simulink model "GNSS_INS"  (R2019b)
settings: Solver=ode3  StartTime=0.0  StopTime=60.0  FixedStep=0.01  RelTol=1e-3
PreLoadFcn:
  | %% SETUP
  | % Start or connect to ROS master
  | rosshutdown;
  | rosinit()
undefined symbols (not defined in the file): Pose, Twist
libraries: robotlib x5
settings Model: Creator=adity  LastModifiedBy=adity
settings OptimizationCC: EnhancedBackFolding=on  PassReuseOutputArgsAs=Individual arguments  ZeroExternalMemoryAtStartup=off  ZeroInternalMemoryAtStartup=off  MaxStackSize=64  OptimizeBlockOrder=speed  DifferentSizesBufferReuse=on  OptimizationCustomize=off  EfficientTunableParamExpr=on
settings DebuggingCC: ParameterTunabilityLossMsg=error
settings HardwareCC: ProdBitPerPointer=32  ProdBitPerSizeT=32  ProdBitPerPtrDiffT=32  ProdLargestAtomicFloat=None  ProdIntDivRoundTo=Undefined  ProdEndianess=Unspecified  ProdWordSize=32  ProdHWDeviceType=Generic->Unspecified (assume 32-bit Generic)  UseEmbeddedCoderFeatures=off
settings SFSimCC: MATLABDynamicMemAlloc=off
settings RTWCC: SystemTargetFile=ert.tlc  HardwareBoard=Robot Operating System (ROS)  TLCOptions="-aInlineSetEventsForThisBaseRateFcn=TLC_FALSE -aSuppressMultiTaskScheduler=TLC_FALSE  -aRateBasedStepFcn=0"  TemplateMakefile=ert_default_tmf  GenerateReport=on  Toolchain=Catkin  IncludeHyperlinkInReport=on  LaunchReport=on  TargetLang=C++  GenerateTraceInfo=on  GenerateTraceReport=on  GenerateTraceReportSl=on  GenerateTraceReportSf=on  GenerateTraceReportEml=on
settings CodeAppCC: ForceParamTrailComments=on  IgnoreCustomStorageClasses=off  OperatorAnnotations=on  SimulinkDataObjDesc=on  SFDataObjDesc=on  InsertBlockDesc=on
settings ERTTargetCC: SupportNonInlinedSFcns=on

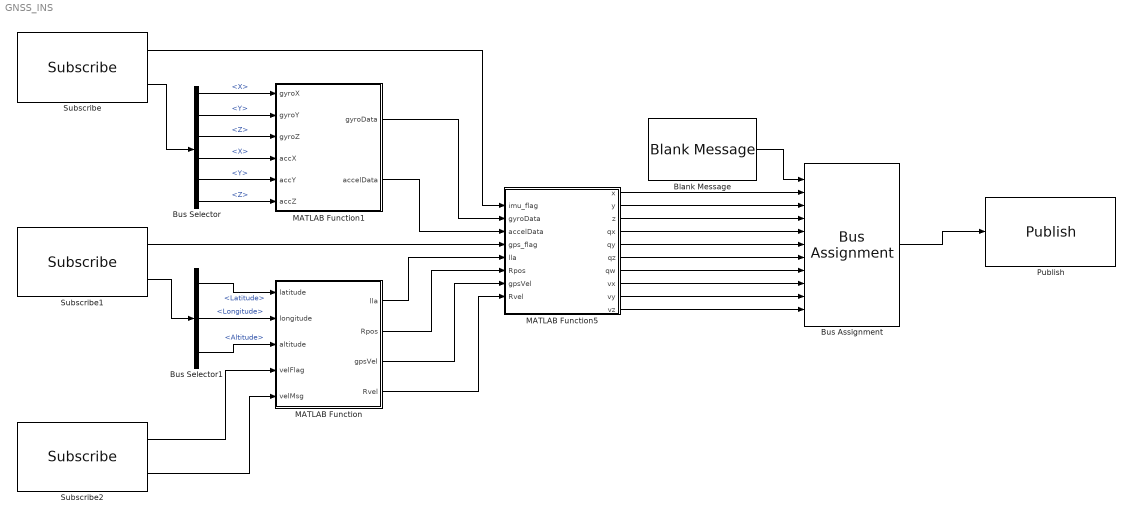
== system GNSS_INS ==
  Blank Message : robotlib/Blank Message  messageClass=Message  entityType=nav_msgs/Odometry  messageType=nav_msgs/Odometry  SampleTime=inf
      settings: SourceProductName=ROS Toolbox
  Bus Assignment : BusAssignment  AssignedSignals=Pose.Pose.Position.X,Pose.Pose.Position.Y,Pose.Pose.Position.Z,Pose.Pose.Orientation.X,Pose.Pose.Orientation.Y,Pose.Pose.Orientation.Z,Pose.Pose.Orientation.W,Twist.Twist.Linear.X,Twist.Twist.Linear.Y,Twist.Twist.Linear.Z
  Bus Selector : BusSelector  OutputSignals=AngularVelocity.X,AngularVelocity.Y,AngularVelocity.Z,LinearAcceleration.X,LinearAcceleration.Y,LinearAcceleration.Z
  Bus Selector1 : BusSelector  OutputSignals=Latitude,Longitude,Altitude
  MATLAB Function : MATLAB Function  TreatAsAtomicUnit=on
  MATLAB Function1 : MATLAB Function  TreatAsAtomicUnit=on
  MATLAB Function5 : MATLAB Function  TreatAsAtomicUnit=on
  Publish : robotlib/Publish  topicSource=Specify your own  topic=/gnss_ins_odom  messageType=nav_msgs/Odometry  messageQueueLength=10
      settings: SourceProductName=ROS Toolbox
  Subscribe : robotlib/Subscribe  topicSource=Select from ROS network  topic=/imu_data  messageType=sensor_msgs/Imu  sampleTime=-1  messageQueueLength=10
      settings: SourceProductName=ROS Toolbox
  Subscribe1 : robotlib/Subscribe  topicSource=Select from ROS network  topic=/fix  messageType=sensor_msgs/NavSatFix  sampleTime=-1  messageQueueLength=10
      settings: SourceProductName=ROS Toolbox
  Subscribe2 : robotlib/Subscribe  topicSource=Select from ROS network  topic=/vel  messageType=geometry_msgs/Vector3Stamped  sampleTime=-1  messageQueueLength=10
      settings: SourceProductName=ROS Toolbox
  wires:
  Subscribe/2 -> Bus Selector/1
  Subscribe1/2 -> Bus Selector1/1
  Bus Selector1/1 -> MATLAB Function/1(latitude)  "<Latitude>"
  Bus Selector1/2 -> MATLAB Function/2(longitude)  "<Longitude>"
  Bus Selector1/3 -> MATLAB Function/3(altitude)  "<Altitude>"
  Bus Selector/1 -> MATLAB Function1/1(gyroX)  "<X>"
  Bus Selector/2 -> MATLAB Function1/2(gyroY)  "<Y>"
  Bus Selector/3 -> MATLAB Function1/3(gyroZ)  "<Z>"
  Bus Selector/4 -> MATLAB Function1/4(accX)  "<X>"
  Bus Selector/5 -> MATLAB Function1/5(accY)  "<Y>"
  Bus Selector/6 -> MATLAB Function1/6(accZ)  "<Z>"
  MATLAB Function1/1(gyroData) -> MATLAB Function5/2(gyroData)
  MATLAB Function1/2(accelData) -> MATLAB Function5/3(accelData)
  MATLAB Function/1(lla) -> MATLAB Function5/5(lla)
  Subscribe1/1 -> MATLAB Function5/4(gps_flag)
  Subscribe/1 -> MATLAB Function5/1(imu_flag)
  MATLAB Function/2(Rpos) -> MATLAB Function5/6(Rpos)
  MATLAB Function/3(gpsVel) -> MATLAB Function5/7(gpsVel)
  MATLAB Function/4(Rvel) -> MATLAB Function5/8(Rvel)
  Blank Message/1 -> Bus Assignment/1
  Bus Assignment/1 -> Publish/1
  MATLAB Function5/1(x) -> Bus Assignment/2
  MATLAB Function5/2(y) -> Bus Assignment/3
  MATLAB Function5/3(z) -> Bus Assignment/4
  MATLAB Function5/4(qx) -> Bus Assignment/5
  MATLAB Function5/5(qy) -> Bus Assignment/6
  MATLAB Function5/6(qz) -> Bus Assignment/7
  MATLAB Function5/7(qw) -> Bus Assignment/8
  MATLAB Function5/8(vx) -> Bus Assignment/9
  MATLAB Function5/9(vy) -> Bus Assignment/10
  MATLAB Function5/10(vz) -> Bus Assignment/11
  Subscribe2/2 -> MATLAB Function/5(velMsg)
  Subscribe2/1 -> MATLAB Function/4(velFlag)

== matlab function GNSS_INS/MATLAB Function1 ==
  data: gyroX input; gyroData output; gyroY input; gyroZ input; accX input; accY input; accZ input; accelData output
function [gyroData, accelData]= imuData(gyroX,gyroY,gyroZ,accX,accY,accZ)
    gyroData = [gyroX,gyroY,gyroZ];
    accelData = [accX,accY,-accZ];
end

== matlab function GNSS_INS/MATLAB Function ==
  data: latitude input; lla output; longitude input; altitude input; velFlag input; Rpos output; gpsVel output; Rvel output; velMsg input
function [lla, Rpos, gpsVel, Rvel] = gpsData(latitude, longitude, altitude, velFlag, velMsg)

    persistent robotVel
    if isempty(robotVel)
        robotVel = [0,0,0];
    end
    if(velFlag)
        robotVel = [velMsg.Vector_.X,velMsg.Vector_.Y,velMsg.Vector_.Z];
    end
    % Assemble GPS data in array
    lla = [latitude,longitude,altitude];
    gpsVel = robotVel;
    % Measurement noises
    Rvel = 0.01;
    Rpos = 0;
end

== matlab function GNSS_INS/MATLAB Function5 ==
  data: imu_flag input; gyroData input; accelData input; gps_flag input; lla input; Rpos input; gpsVel input; Rvel input; x output; y output; z output; qx output; qy output; qz output; qw output; vx output; vy output; vz output
function [x,y,z,qx,qy,qz,qw,vx,vy,vz]= fuseIMUGPS(imu_flag, gyroData, accelData, gps_flag, lla, Rpos, gpsVel, Rvel)
    persistent gndFusion
    if isempty(gndFusion)
        imuFs = 50;
        localOrigin = [18.954817 72.811367 0];

        gndFusion = insfilterNonholonomic('ReferenceFrame', 'ENU', ...
            'IMUSampleRate', imuFs, ...
            'ReferenceLocation', localOrigin, ...
            'DecimationFactor', 2);

        % Initialize the states of the filter
        gndFusion.State(1:4) = [0.707,0,0,0.707];
        gndFusion.State(5:7) = [0,0,0];
        gndFusion.State(8:10) = [0,0,0];
        gndFusion.State(11:13) = [0,0,0];
        gndFusion.State(14:16) = [0,0,0];

        % |ZeroVelocityConstraintNoise| parameter.
        gndFusion.ZeroVelocityConstraintNoise = 1e-2;

        % Process noises
        gndFusion.GyroscopeNoise = 2.5e-5;
        gndFusion.GyroscopeBiasNoise = 1.4e-8;
        gndFusion.AccelerometerNoise = 2.5e-5;
        gndFusion.AccelerometerBiasNoise = 1.4e-8;

        % Initial error covariance
        gndFusion.StateCovariance = 1e-9*ones(16);
    end
    
    if(imu_flag)
        predict(gndFusion, accelData, gyroData);
    end
    
    if(gps_flag)
        fusegps(gndFusion, lla, Rpos, gpsVel, Rvel);
    end
    
    [pos,or,vel] = pose(gndFusion);
    temp = compact(or);
    x = pos(1);
    y = pos(2);
    z = pos(3);
    qw = temp(1);
    qx = temp(2);
    qy = temp(3);
    qz = temp(4);
    vx = vel(1);
    vy = vel(2);
    vz = vel(3);
    
end
